simulink model "newsyscase1mod"  (R2014b)
settings: Solver=ode45  StartTime=0.0  StopTime=1000  RelTol=1e-3
undefined symbols (not defined in the file or in its folder): u1, u2, u3, u4
undefined symbols (not defined in the file): H1C1initT, H1C2initT, H2C1initT, H2C2initT, H2C3initT, Ttank1, Ttank2, Ttank3, Ttank4, Ttank5
settings Model: Creator=fredrik  LastModifiedBy=fredrik

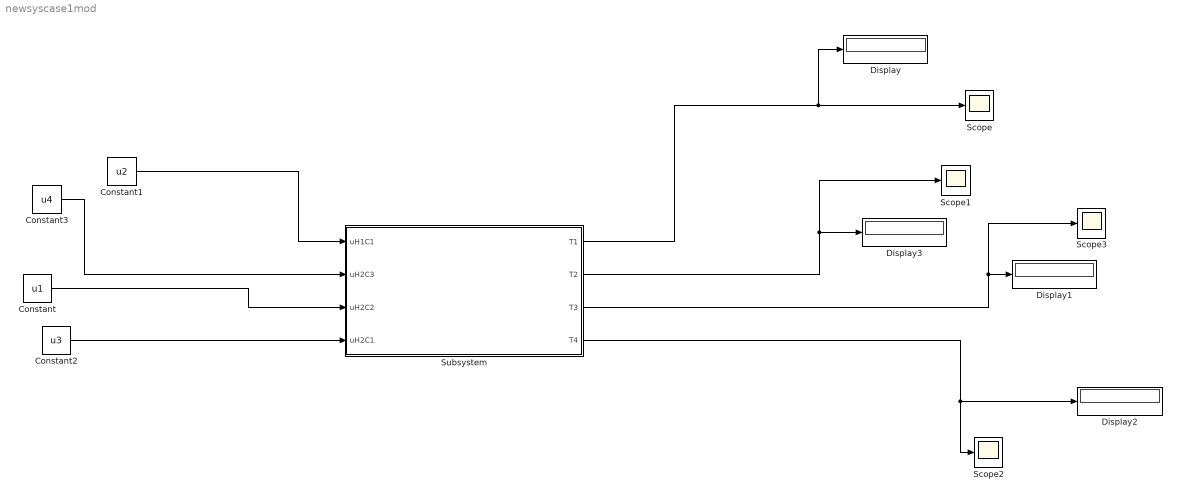
== system newsyscase1mod ==
  Constant : Constant  Value=u1
  Constant1 : Constant  Value=u2
  Constant2 : Constant  Value=u3
  Constant3 : Constant  Value=u4
  Display{,1..3} (4 alike) : Display
  Scope{,1..3} (4 alike) : Scope
      Scope settings: YMin=-0  YMax=400
      Scope1 settings: YMin=0  YMax=400
      Scope2 settings: YMin=0  YMax=400  SaveName=ScopeData3
      Scope3 settings: YMin=0  YMax=400  SaveName=ScopeData5
  Subsystem : Subsystem
  wires:
  Subsystem/1(T1) -> Display/1, Scope/1
  Subsystem/3(T3) -> Scope3/1, Display1/1
  Subsystem/4(T4) -> Scope2/1, Display2/1
  Subsystem/2(T2) -> Display3/1, Scope1/1
  Constant2/1 -> Subsystem/4(uH2C1)
  Constant1/1 -> Subsystem/1(uH1C1)
  Constant/1 -> Subsystem/3(uH2C2)
  Constant3/1 -> Subsystem/2(uH2C3)

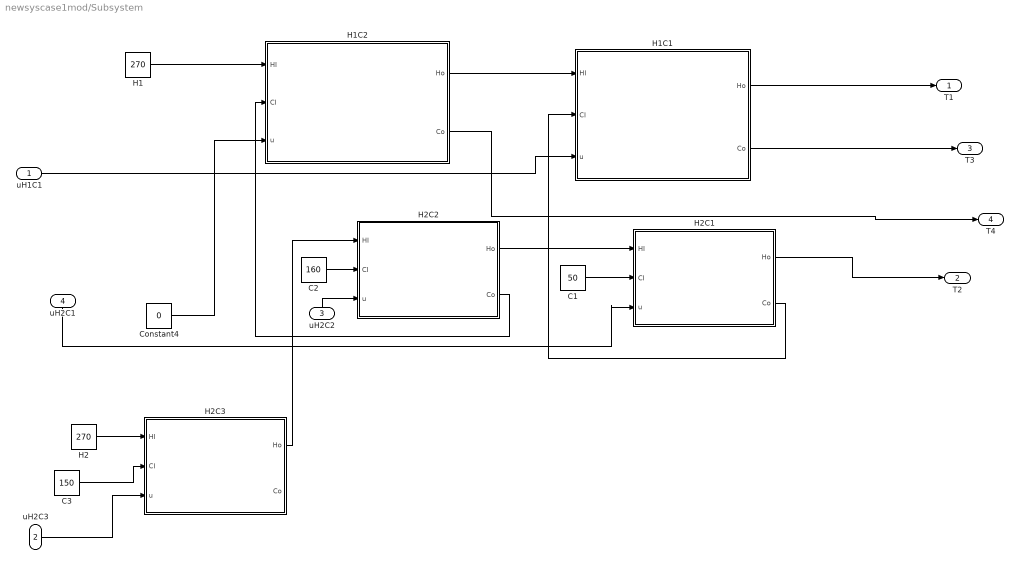
== system newsyscase1mod/Subsystem ==
  uH1C1 : Inport
  uH2C3 : Inport  Port=2
  uH2C2 : Inport  Port=3
  uH2C1 : Inport  Port=4
  C1 : Constant  Value=50
  C2 : Constant  Value=160
  C3 : Constant  Value=150
  Constant4 : Constant  Value=0
  H1 : Constant  Value=270
  H1C1 : Subsystem  mask{A=239.1281493, t=Ttank2, Q=1000, Ulm=0.5, Thin=225.55555, Thout=170, Tcin=160, Tcout=210, n=10, initT=H1C1initT, hot=1}
      mask prompts: A "Area"; t "Time in tank"; Ulm "U"; Thin "Hotin"; Thout "Hotout"; Tcin "Coldin"; Tcout "Coldout"; n "Number of cells"; initT "initial temperature"; hot "1 if hot bypass, 0 if cold"
      mask init:
      | % vH=sym('vH');
      | % Vh=sym('Vh');
      | % th=sym('th');
      | % u0=sym('u0'); %
      | % Vend=sym('Vend');
      | % vC=sym('vC');
      | % Vc=sym('Vc');
      | % tc=sym('tc');
      | 
      | %%tank1:
      | 
      | %% E-2401
      | Fc=Q/(Tcout-Tcin);
      | Fh=Q/(Thin-Thout);
      | Fsak=2*1/(1/Fc+1/Fh);
      | Nth=Ulm*A/Fsak;
      | U=Ulm/(n-Nth)*n;
      | UA=A*U;
      | tc=1/(UA/(Fc*t));%cold constant for transfer
      | th=1/(UA/(Fh*t));%hot constant for transfer
      | A=zeros(2*n+1);
      | AU=zeros(2*n+1);
      | 
      | B=zeros(2*n,1);
      | C=zeros(2,2*n+1);
      | if hot
      |     C(2,end)=1;
      |     C(1,2)=1;
      | else
      |     C(1,end)=1;
      |     C(2,end-2)=1;
      | end
      | D=zeros(2*n,1);
      | 
      | 
      | for k=1:2*n
      |     if mod(k,2) == 1
      |         A(k,k)=-(1/th+n/t);
      |         A(k,k+1)=1/th;
      |         if hot
      |             AU(k,k)=n/t;
      |         end
      |         if k~=1
      |             A(k,k-2)=n/t;
      |             if hot
      |                 AU(k,k-2)=-n/t;
      |             end
      |         end
      |     else
      |         A(k,k)=-(n/t+1/tc);
      |         A(k,k-1)=1/tc;
      |         if ~hot
      |             AU(k,k)=n/t;
      |         end
      |         if k~=2*n
      |             A(k,k+2)=n/t;
      |             if ~hot
      |                 AU(k,k+2)=-n/t;
      |             end
      |         end
      |     end
      | end
      | Ds=zeros(2*n+1,2);
      | %Ds=sym(Ds);
      | Ds(1,1)=(n/t);
      | Ds(2*n,2)=(n/t);
      | DsU=zeros(2*n+1,2);
      | %DsU=sym(DsU);
      | if hot
      |     DsU(1,1)=(-n/t);
      | else
      |     DsU(2*n,2)=(-n/t);
      | end
      | 
      | 
      | if hot
      |     A(2*n+1,end-2)=n/t;
      |     AU(2*n+1,end-2)=-n/t;
      |     A(2*n+1,end)=-n/t;
      |     DsU(end,1)=n/t;
      | else
      |     A(2*n+1,2)=n/t;
      |     A(2*n+1,end)=-n/t;
      |     AU(2*n+1,2)=-n/t;
      |     DsU(end,2)=n/t;
      | end
      | %DsU(end,1)=1;
      | %A(2*n+1,end-2)=1;
      | %AU(2*n+1,end-2)=-1;
      | 
      | 
      | 
      | % x=zeroes(10000,2*n);
      | % k=0:0.1:1000;
      | % X=zeroes(10000,2*n);
      | % X(1,:)=initT;
      | % for k=0:1:10000;
      | %
      | % end
      | %
      | % X=A*X+Ds*TI;
      | 
      | 
      | %A=[-(3*vH/Vh*(1-u0)+1/th) 1/th 0 0 0 0 0; 1/tc -(3*vC/Vc+1/tc) 0 3*vC/Vc 0 0 0; 3*vH/Vh*(1-u0) 0 -(3*vH/Vh*(1-u0)+1/th) 1/th 0 0 0; 0 0 1/tc -(3*vC/Vc+1/tc) 0 3*vC/Vc 0;0 0 3*vH/Vh*(1-u0) 0 -(3*vH/Vh*(1-u0)+1/th) 1/th 0;0 0 0 0 1/tc -(3*vC/Vc+1/tc) 0; 0 0 0 0 (1-u0)*vH/Vend 0 -vH/Vend];A
  H1C2 : Subsystem  mask{A=28.27287318, t=Ttank1, Q=800, Ulm=0.5, Thin=270, Thout=225.5555, Tcin=182, Tcout=198, n=10, initT=H1C2initT, hot=1}
      mask prompts: A "Area"; t "Time in tank"; Ulm "U"; Thin "Hotin"; Thout "Hotout"; Tcin "Coldin"; Tcout "Coldout"; n "Number of cells"; initT "initial temperature"; hot "1 if hot bypass, 0 if cold"
      mask init: same as newsyscase1mod/Subsystem/H1C1
  H2 : Constant  Value=270
  H2C1 : Subsystem  mask{A=466.4208212, t=Ttank4, Q=2200, Ulm=0.5, Thin=170, Thout=70, Tcin=50, Tcout=160, n=15, initT=H2C1initT, hot=1}
      mask prompts: A "Area"; t "Time in tank"; Ulm "U"; Thin "Hotin"; Thout "Hotout"; Tcin "Coldin"; Tcout "Coldout"; n "Number of cells"; initT "initial temperature"; hot "1 if hot bypass, 0 if cold"
      mask init: same as newsyscase1mod/Subsystem/H1C1
  H2C2 : Subsystem  mask{A=140.693508, t=Ttank3, Q=1100, Ulm=0.5, Thin=220, Thout=170, Tcin=160, Tcout=182, n=10, initT=H2C2initT, hot=1}
      mask prompts: A "Area"; t "Time in tank"; Ulm "U"; Thin "Hotin"; Thout "Hotout"; Tcin "Coldin"; Tcout "Coldout"; n "Number of cells"; initT "initial temperature"; hot "1 if hot bypass, 0 if cold"
      mask init: same as newsyscase1mod/Subsystem/H1C1
  H2C3 : Subsystem  mask{A=57.91852701, t=Ttank5, Q=1100, Ulm=0.5, Thin=270, Thout=220, Tcin=150, Tcout=250, n=10, initT=H2C3initT, hot=1}
      mask prompts: A "Area"; t "Time in tank"; Ulm "U"; Thin "Hotin"; Thout "Hotout"; Tcin "Coldin"; Tcout "Coldout"; n "Number of cells"; initT "initial temperature"; hot "1 if hot bypass, 0 if cold"
      mask init: same as newsyscase1mod/Subsystem/H1C1
  T1 : Outport
  T2 : Outport  Port=2
  T3 : Outport  Port=3
  T4 : Outport  Port=4
  wires:
  H2C1/1(Ho) -> T2/1
  H1C1/2(Co) -> T3/1
  H2C2/2(Co) -> H1C2/2(CI)
  H1C1/1(Ho) -> T1/1
  uH2C1/1 -> H2C1/3(u)
  uH1C1/1 -> H1C1/3(u)
  H1/1 -> H1C2/1(HI)
  C1/1 -> H2C1/2(CI)
  C2/1 -> H2C2/2(CI)
  H2/1 -> H2C3/1(HI)
  C3/1 -> H2C3/2(CI)
  uH2C3/1 -> H2C3/3(u)
  H1C2/1(Ho) -> H1C1/1(HI)
  H2C3/1(Ho) -> H2C2/1(HI)
  H1C2/2(Co) -> T4/1
  Constant4/1 -> H1C2/3(u)
  uH2C2/1 -> H2C2/3(u)
  H2C2/1(Ho) -> H2C1/1(HI)
  H2C1/2(Co) -> H1C1/2(CI)

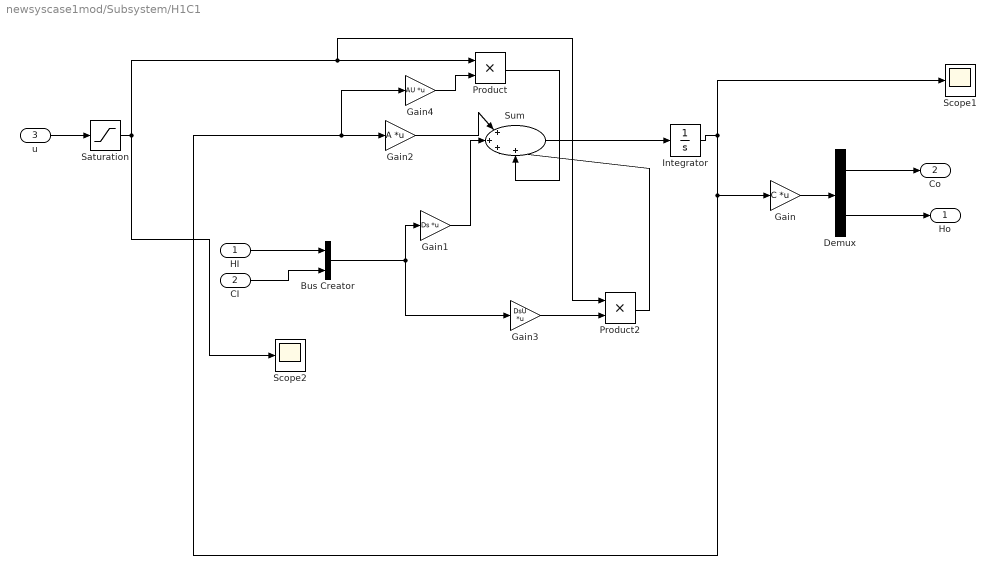
== system newsyscase1mod/Subsystem/H1C1 ==
  HI : Inport
  CI : Inport  Port=2
  u : Inport  Port=3
  Bus Creator : BusCreator  Inputs=2
  Demux : Demux  Outputs=2
  Gain : Gain  Gain=C  Multiplication=Matrix(K*u)
  Gain1 : Gain  Gain=Ds  Multiplication=Matrix(K*u)
  Gain2 : Gain  Gain=A  Multiplication=Matrix(K*u)
  Gain3 : Gain  Gain=DsU  Multiplication=Matrix(K*u)
  Gain4 : Gain  Gain=AU  Multiplication=Matrix(K*u)
  Integrator : Integrator  InitialCondition=initT
  Product : Product
  Product2 : Product
  Saturation : Saturate  UpperLimit=1  LowerLimit=0
  Scope1 : Scope
      settings: ShowLegends=on  YMin=60  YMax=220  SaveName=ScopeData4
  Scope2 : Scope
      settings: SaveName=ScopeData2
  Sum : Sum  Inputs=|++++
  Ho : Outport
  Co : Outport  Port=2
  wires:
  Integrator/1 -> Gain4/1, Gain2/1, Gain/1, Scope1/1
  Sum/1 -> Integrator/1
  Gain2/1 -> Sum/1
  Bus Creator/1 -> Gain1/1, Gain3/1
  Gain1/1 -> Sum/2
  Product/1 -> Sum/4
  Gain3/1 -> Product2/2
  Product2/1 -> Sum/3
  Gain4/1 -> Product/2
  Saturation/1 -> Product2/1, Product/1, Scope2/1
  HI/1 -> Bus Creator/1
  CI/1 -> Bus Creator/2
  Demux/2 -> Ho/1
  Demux/1 -> Co/1
  Gain/1 -> Demux/1
  u/1 -> Saturation/1

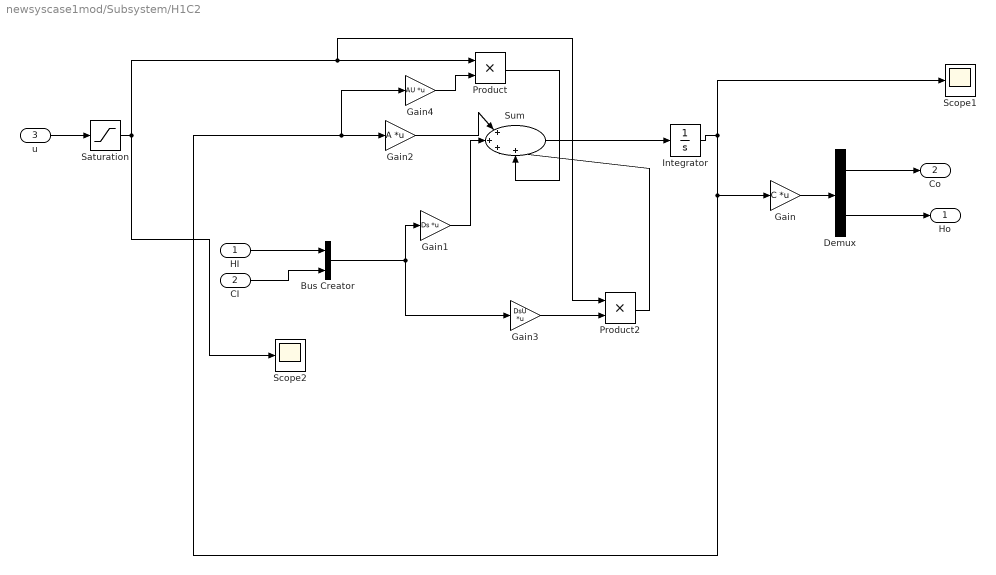
== system newsyscase1mod/Subsystem/H1C2 ==
  HI : Inport
  CI : Inport  Port=2
  u : Inport  Port=3
  Bus Creator : BusCreator  Inputs=2
  Demux : Demux  Outputs=2
  Gain : Gain  Gain=C  Multiplication=Matrix(K*u)
  Gain1 : Gain  Gain=Ds  Multiplication=Matrix(K*u)
  Gain2 : Gain  Gain=A  Multiplication=Matrix(K*u)
  Gain3 : Gain  Gain=DsU  Multiplication=Matrix(K*u)
  Gain4 : Gain  Gain=AU  Multiplication=Matrix(K*u)
  Integrator : Integrator  InitialCondition=initT
  Product : Product
  Product2 : Product
  Saturation : Saturate  UpperLimit=1  LowerLimit=0
  Scope1 : Scope
      settings: ShowLegends=on  YMin=60  YMax=220  SaveName=ScopeData4
  Scope2 : Scope
      settings: SaveName=ScopeData2
  Sum : Sum  Inputs=|++++
  Ho : Outport
  Co : Outport  Port=2
  wires:
  Integrator/1 -> Gain4/1, Gain2/1, Gain/1, Scope1/1
  Sum/1 -> Integrator/1
  Gain2/1 -> Sum/1
  Bus Creator/1 -> Gain1/1, Gain3/1
  Gain1/1 -> Sum/2
  Product/1 -> Sum/4
  Gain3/1 -> Product2/2
  Product2/1 -> Sum/3
  Gain4/1 -> Product/2
  Saturation/1 -> Product2/1, Product/1, Scope2/1
  HI/1 -> Bus Creator/1
  CI/1 -> Bus Creator/2
  Demux/2 -> Ho/1
  Demux/1 -> Co/1
  Gain/1 -> Demux/1
  u/1 -> Saturation/1

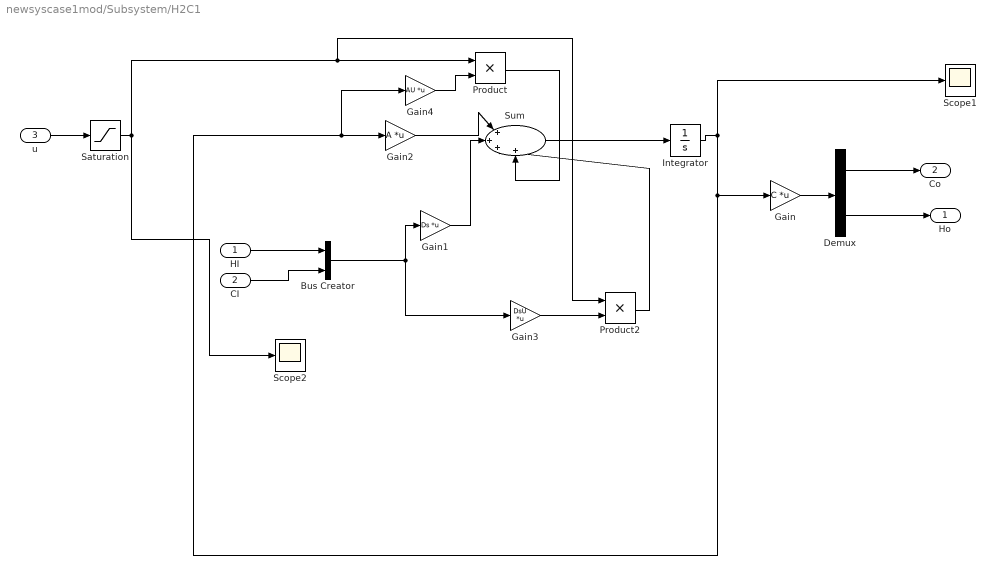
== system newsyscase1mod/Subsystem/H2C1 ==
  HI : Inport
  CI : Inport  Port=2
  u : Inport  Port=3
  Bus Creator : BusCreator  Inputs=2
  Demux : Demux  Outputs=2
  Gain : Gain  Gain=C  Multiplication=Matrix(K*u)
  Gain1 : Gain  Gain=Ds  Multiplication=Matrix(K*u)
  Gain2 : Gain  Gain=A  Multiplication=Matrix(K*u)
  Gain3 : Gain  Gain=DsU  Multiplication=Matrix(K*u)
  Gain4 : Gain  Gain=AU  Multiplication=Matrix(K*u)
  Integrator : Integrator  InitialCondition=initT
  Product : Product
  Product2 : Product
  Saturation : Saturate  UpperLimit=1  LowerLimit=0
  Scope1 : Scope
      settings: ShowLegends=on  YMin=60  YMax=220  SaveName=ScopeData4
  Scope2 : Scope
      settings: SaveName=ScopeData2
  Sum : Sum  Inputs=|++++
  Ho : Outport
  Co : Outport  Port=2
  wires:
  Integrator/1 -> Gain4/1, Gain2/1, Gain/1, Scope1/1
  Sum/1 -> Integrator/1
  Gain2/1 -> Sum/1
  Bus Creator/1 -> Gain1/1, Gain3/1
  Gain1/1 -> Sum/2
  Product/1 -> Sum/4
  Gain3/1 -> Product2/2
  Product2/1 -> Sum/3
  Gain4/1 -> Product/2
  Saturation/1 -> Product2/1, Product/1, Scope2/1
  HI/1 -> Bus Creator/1
  CI/1 -> Bus Creator/2
  Demux/2 -> Ho/1
  Demux/1 -> Co/1
  Gain/1 -> Demux/1
  u/1 -> Saturation/1

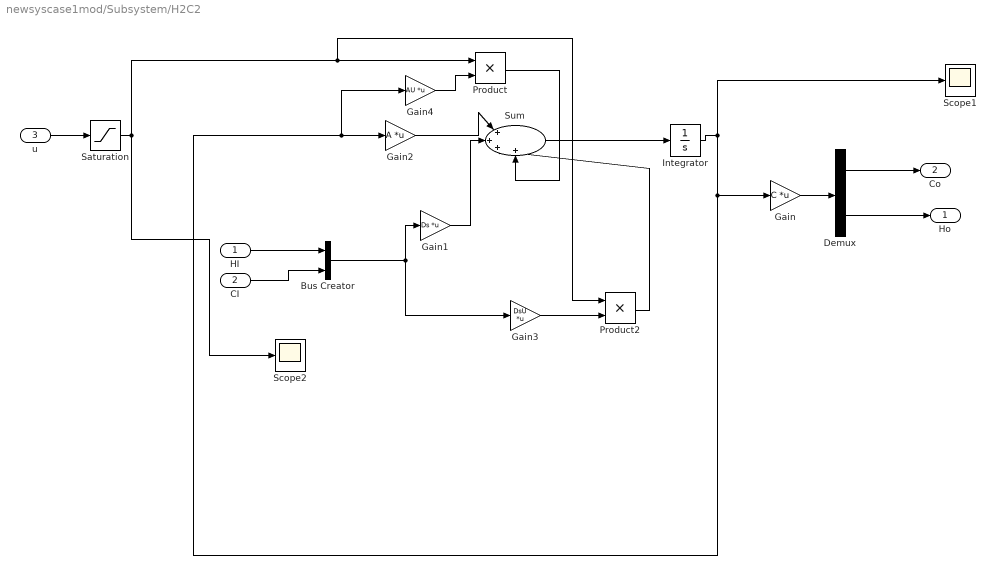
== system newsyscase1mod/Subsystem/H2C2 ==
  HI : Inport
  CI : Inport  Port=2
  u : Inport  Port=3
  Bus Creator : BusCreator  Inputs=2
  Demux : Demux  Outputs=2
  Gain : Gain  Gain=C  Multiplication=Matrix(K*u)
  Gain1 : Gain  Gain=Ds  Multiplication=Matrix(K*u)
  Gain2 : Gain  Gain=A  Multiplication=Matrix(K*u)
  Gain3 : Gain  Gain=DsU  Multiplication=Matrix(K*u)
  Gain4 : Gain  Gain=AU  Multiplication=Matrix(K*u)
  Integrator : Integrator  InitialCondition=initT
  Product : Product
  Product2 : Product
  Saturation : Saturate  UpperLimit=1  LowerLimit=0
  Scope1 : Scope
      settings: ShowLegends=on  YMin=60  YMax=220  SaveName=ScopeData4
  Scope2 : Scope
      settings: SaveName=ScopeData2
  Sum : Sum  Inputs=|++++
  Ho : Outport
  Co : Outport  Port=2
  wires:
  Integrator/1 -> Gain4/1, Gain2/1, Gain/1, Scope1/1
  Sum/1 -> Integrator/1
  Gain2/1 -> Sum/1
  Bus Creator/1 -> Gain1/1, Gain3/1
  Gain1/1 -> Sum/2
  Product/1 -> Sum/4
  Gain3/1 -> Product2/2
  Product2/1 -> Sum/3
  Gain4/1 -> Product/2
  Saturation/1 -> Product2/1, Product/1, Scope2/1
  HI/1 -> Bus Creator/1
  CI/1 -> Bus Creator/2
  Demux/2 -> Ho/1
  Demux/1 -> Co/1
  Gain/1 -> Demux/1
  u/1 -> Saturation/1

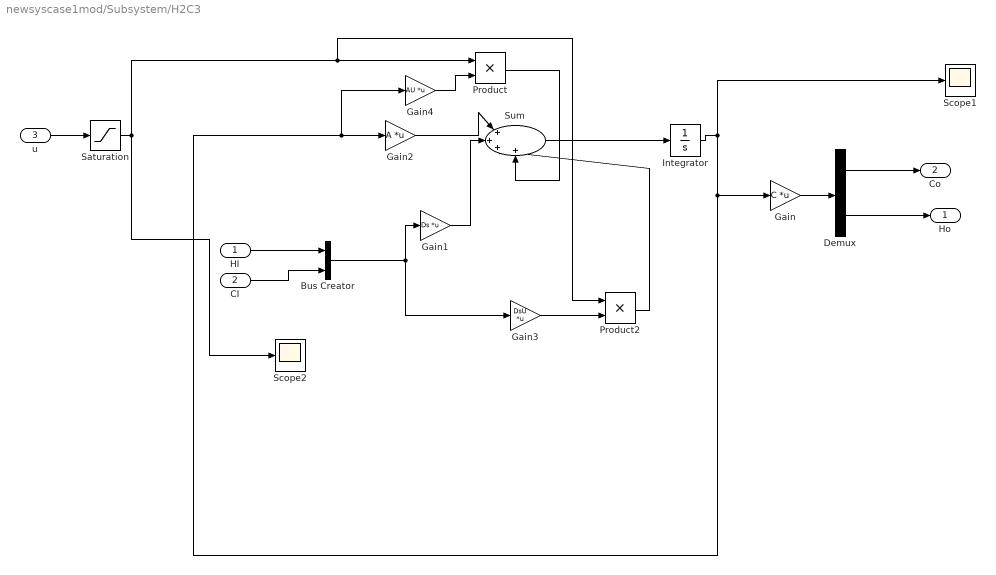
== system newsyscase1mod/Subsystem/H2C3 ==
  HI : Inport
  CI : Inport  Port=2
  u : Inport  Port=3
  Bus Creator : BusCreator  Inputs=2
  Demux : Demux  Outputs=2
  Gain : Gain  Gain=C  Multiplication=Matrix(K*u)
  Gain1 : Gain  Gain=Ds  Multiplication=Matrix(K*u)
  Gain2 : Gain  Gain=A  Multiplication=Matrix(K*u)
  Gain3 : Gain  Gain=DsU  Multiplication=Matrix(K*u)
  Gain4 : Gain  Gain=AU  Multiplication=Matrix(K*u)
  Integrator : Integrator  InitialCondition=initT
  Product : Product
  Product2 : Product
  Saturation : Saturate  UpperLimit=1  LowerLimit=0
  Scope1 : Scope
      settings: ShowLegends=on  YMin=60  YMax=220  SaveName=ScopeData4
  Scope2 : Scope
      settings: SaveName=ScopeData2
  Sum : Sum  Inputs=|++++
  Ho : Outport
  Co : Outport  Port=2
  wires:
  Integrator/1 -> Gain4/1, Gain2/1, Gain/1, Scope1/1
  Sum/1 -> Integrator/1
  Gain2/1 -> Sum/1
  Bus Creator/1 -> Gain1/1, Gain3/1
  Gain1/1 -> Sum/2
  Product/1 -> Sum/4
  Gain3/1 -> Product2/2
  Product2/1 -> Sum/3
  Gain4/1 -> Product/2
  Saturation/1 -> Product2/1, Product/1, Scope2/1
  HI/1 -> Bus Creator/1
  CI/1 -> Bus Creator/2
  Demux/2 -> Ho/1
  Demux/1 -> Co/1
  Gain/1 -> Demux/1
  u/1 -> Saturation/1
